simulink model "full_order_observer_controller_simulation"  (R2016a)
settings: Solver=VariableStepAuto  StartTime=0.0  StopTime=20.0  RelTol=1e-3
values from neighbouring files (symbols this model uses):
  a = obj.a    [System.m]    (also in system_examples.m = [-15,-14,-24;-14,-14,-24;15,15,25])
  b = obj.b    [System.m]    (also in system_examples.m = [1;1;-1])
  c = obj.c    [System.m]    (also in system_examples.m = [1,1,2])
  css = eye(size(a))    [System.m]
  dss = [zeros(size(a,1), 1)]    [System.m]
  k = place(an, bn, des_eigs)    [System.m]    (also in system_examples.m = ol_sys.get_control_gain(des_poles))
  l = obj.full_observer_gain(des_eigs)    [System.m]
  x0 = obj.x0    [System.m]
settings Model: Creator=micah  LastModifiedBy=micah

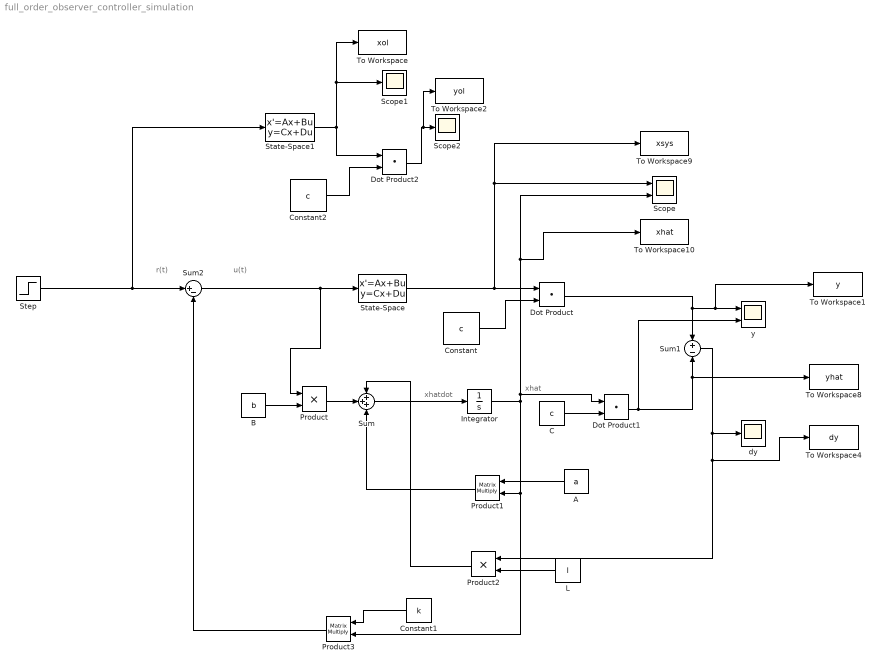
== system full_order_observer_controller_simulation ==
  note: r(t)
  note: u(t)
  note: xhatdot
  note: xhat
  A : Constant  Value=a  VectorParams1D=off
  B : Constant  Value=b  VectorParams1D=off
  C : Constant  Value=c  VectorParams1D=off
  Constant : Constant  Value=c
  Constant1 : Constant  Value=k  VectorParams1D=off
  Constant2 : Constant  Value=c
  Dot Product : DotProduct  InputSameDT=on  OutDataTypeStr=Inherit: Inherit via internal rule
  Dot Product1 : DotProduct  InputSameDT=on  OutDataTypeStr=Inherit: Inherit via internal rule
  Dot Product2 : DotProduct  InputSameDT=on  OutDataTypeStr=Inherit: Inherit via internal rule
  Integrator : Integrator  InitialCondition=zeros(size(b))
  "L " : Constant  Value=l
  Product : Product
  Product1 : Product  Multiplication=Matrix(*)
  Product2 : Product
  Product3 : Product  Multiplication=Matrix(*)
  Scope : Scope  NumInputPorts=2
  Scope1 : Scope
  Scope2 : Scope
  State-Space : StateSpace  A=a  B=b  C=css  D=dss  X0=x0
  State-Space1 : StateSpace  A=a  B=b  C=css  D=dss  X0=x0
  Step : Step  Time=0  SampleTime=0
  Sum : Sum  Inputs=+++
  Sum1 : Sum  Inputs=+-
  Sum2 : Sum  Inputs=|+-
  To Workspace : ToWorkspace  VariableName=xol  SaveFormat=Structure With Time  SampleTime=-1
  To Workspace1 : ToWorkspace  VariableName=y  SaveFormat=Structure With Time  SampleTime=-1
  To Workspace10 : ToWorkspace  VariableName=xhat  SaveFormat=Structure With Time  SampleTime=-1
  To Workspace2 : ToWorkspace  VariableName=yol  SaveFormat=Structure With Time  SampleTime=-1
  To Workspace4 : ToWorkspace  VariableName=dy  SaveFormat=Structure With Time  SampleTime=-1
  To Workspace8 : ToWorkspace  VariableName=yhat  SaveFormat=Structure With Time  SampleTime=-1
  To Workspace9 : ToWorkspace  VariableName=xsys  SaveFormat=Structure With Time  SampleTime=-1
  dy : Scope
  y : Scope  NumInputPorts=2
  wires:
  Sum2/1 -> Product/1, State-Space/1
  State-Space/1 -> To Workspace9/1, Scope/1, Dot Product/1
  Constant/1 -> Dot Product/2
  Dot Product/1 -> Sum1/1, To Workspace1/1, y/1
  B/1 -> Product/2
  Product/1 -> Sum/2
  Sum/1 -> Integrator/1
  A/1 -> Product1/1
  Product1/1 -> Sum/3
  C/1 -> Dot Product1/2
  Dot Product1/1 -> y/2, Sum1/2, To Workspace8/1
  Sum1/1 -> To Workspace4/1, Product2/1, dy/1
  "L "/1 -> Product2/2
  Product2/1 -> Sum/1
  Integrator/1 -> Scope/2, To Workspace10/1, Dot Product1/1, Product3/2, Product1/2
  Constant1/1 -> Product3/1
  Step/1 -> State-Space1/1, Sum2/1
  Product3/1 -> Sum2/2
  State-Space1/1 -> Dot Product2/1, To Workspace/1, Scope1/1
  Constant2/1 -> Dot Product2/2
  Dot Product2/1 -> To Workspace2/1, Scope2/1
